simulink model "Example_3_Unregulated_SFR"  (Simulink 8.9)
settings: Solver=VariableStepAuto  StartTime=0.0  StopTime=100  RelTol=1e-3
settings Model: Creator=Prof Francisco Gonzalez-Longatt  LastModifiedBy=fglon
settings DataIOCC: LimitDataPoints=off  SaveFormat=Dataset  SignalLoggingSaveFormat=Dataset  ReturnWorkspaceOutputs=on
settings OptimizationCC: LifeSpan=auto
settings DebuggingCC: UnderspecifiedInitializationDetection=Simplified  MergeDetectMultiDrivingBlocksExec=error  FcnCallInpInsideContextMsg=error  StateNameClashWarn=none  SFUnexpectedBacktrackingDiag=error  SFNoUnconditionalDefaultTransitionDiag=error  SFExecutionAtInitializationDiag=warning
settings HardwareCC: ProdBitPerPointer=64  ProdBitPerSizeT=64  ProdBitPerPtrDiffT=64  ProdLargestAtomicFloat=Float  ProdIntDivRoundTo=Zero  ProdEndianess=LittleEndian  ProdWordSize=64  ProdHWDeviceType=Intel->x86-64 (Windows64)
settings ModelReferenceCC: PropagateSignalLabelsOutOfModel=on
settings SFSimCC: SimUseLocalCustomCode=on
settings RTWCC: RTWUseLocalCustomCode=on
settings GRTTargetCC: TargetLangStandard=C99 (ISO)  CombineOutputUpdateFcns=on  GRTInterface=off
settings ConfigComp: CovMetricSettings=dwe  CovHtmlReporting=off  CovSaveCumulativeToWorkspaceVar=off  CovSaveSingleToWorkspaceVar=off  CovExternalEMLEnable=on

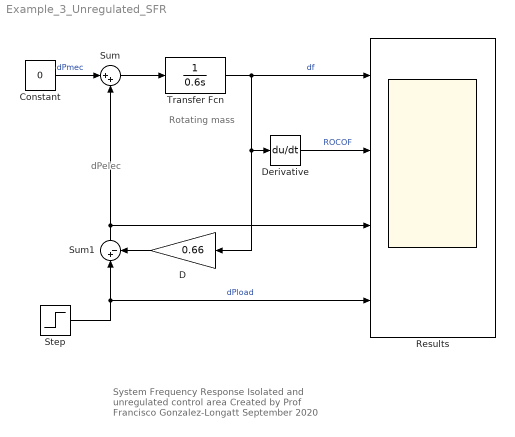
== system Example_3_Unregulated_SFR ==
  note: Rotating mass
  note: System Frequency Response
      | Isolated and unregulated control area
      | Created by Prof  Francisco Gonzalez-Longatt
      | September 2020
  note: dPelec
  Constant : Constant  Value=0
  D : Gain  Gain=0.66
  Derivative : Derivative
  Results : Scope  NumInputPorts=4
  Step : Step  After=-0.05  SampleTime=0
  Sum : Sum  Inputs=|++
  Sum1 : Sum  Inputs=|+-
  Transfer Fcn : TransferFcn  Denominator=[0.6 0]
  wires:
  Sum/1 -> Transfer Fcn/1
  Constant/1 -> Sum/1  "dPmec"
  Sum1/1 -> Sum/2, Results/3
  Step/1 -> Sum1/1, Results/4  "dPload"
  Transfer Fcn/1 -> D/1, Derivative/1, Results/1  "df"
  D/1 -> Sum1/2
  Derivative/1 -> Results/2  "ROCOF"
